simulink model "WormAndGearConstraint"  (R2024a)
settings: Solver=ode45  StartTime=0.0  StopTime=120  MaxStep=0.01  RelTol=1e-3
PreLoadFcn:
  | addpath(fullfile('WormAndGearConstraintSupport','Data'));
  | addpath(fullfile('WormAndGearConstraintSupport','Scripts'));
model workspace: external: MATLAB File WormAndGearConstraintParameters.m (data not in the file)
undefined symbols (not defined in the file or in its folder): slewdrive, X, Y, Z
libraries: sm_lib x75, neural x40, nesl_utility x38, fl_lib x32, WormAndGearConstraintLibrary x24, ee_lib x6, slpidlib x6, spsSeriesRLCBranchLib x2, fl_ps_legacy_lib x1, spsPWMGeneratorDCDCLib x1, spsMosfetLib x1, spsPVArrayLib x1
(part 1 of 6)
CloseFcn:
  | rmpath(fullfile('WormAndGearConstraintSupport','Data'));
  | rmpath(fullfile('WormAndGearConstraintSupport','Scripts'));
Description:
  | Using the Worm and Gear Constraint Block - Solar Tracker
settings Model: SimulationMode=accelerator  Creator=The MathWorks, Inc.  LastModifiedBy=Kshitij Shetty
settings SolverCC: AlgebraicLoopSolver=TrustRegion
settings DataIOCC: ReturnWorkspaceOutputs=off
settings OptimizationCC: ReuseModelBlockBuffer=off
settings DebuggingCC: UnconnectedInputMsg=warning  UnconnectedOutputMsg=warning  UnconnectedLineMsg=warning  SubsystemReferenceDiagnosticForUnitTest=warning  ArithmeticOperatorsInVariantConditions=warning
settings ModelReferenceCC: EnableRefExpFcnMdlSchedulingChecks=on
settings SFSimCC: SimUseLocalCustomCode=off  CustomCodeUndefinedFunction=UseInterfaceOnly
settings RTWCC: RTWUseLocalCustomCode=off  GPUComputeCapability=3.5
settings CodeAppCC: StateflowObjectComments=on
settings ConfigComp: CovMetricSettings=dswe
settings SimscapeCC: SimscapeNormalizeSystem=off  SimscapeNominalValues="[{\"value\":\"10\",\"unit\":\"V\"},{\"value\":\"1\",\"unit\":\"A\"},{\"value\":\"10\",\"unit\":\"N*m\"},{\"value\":\"10\",\"unit\":\"bar\"},{\"value\":\"100\",\"unit\":\"kJ/kg\"},{\"value\":\"1\",\"unit\":\"kW\"},{\"value\":\"300\",\"unit\":\"K\"},{\"value\":\"100\",\"unit\":\"cm^3/s\"},{\"value\":\"1\",\"unit\":\"kN\"},{\"value\":\"1\",\"unit\":\"g/cm^3\"},{\"value\":\"1\",\"unit\":\"l\"},{\"value\":\"1\",\"unit\":\"cm^2\"},{\"value\":\"60\",\"unit\":\"Hz\"}]"  SimscapeLogType=all  SimscapeLogSimulationStatistics=on  SimscapeLogName=simlogWormAndGearConstraint
settings DiagnosticsConfigSet: SimMechanicsUnconnectedFramePorts=none
settings ExplorerConfigSet: InternalSimMechanicsExplorerSettings="<ExplorerConfiguration><canonicalview>default</canonicalview><AnimationSetting><BasePlaybackSpeed>1.0</BasePlaybackSpeed><PlaybackSpeedFactor>2.0</PlaybackSpeedFactor></AnimationSetting><TilePanel><TileInfo><Tiles Columns=\"1\" Count=\"2\" Rows=\"2\"><Column Weight=\"1\"/><Row Weight=\"0.499\"/><Row Weight=\"0.501\"/><Tile Height=\"1\" Width=\"1\" X=\"0\" Y=\"0\"/><Tile Height=\"1\" Width=\"1\" X=\"0\" Y=\"1\"/></Tiles></TileInfo><SceneInfo><SceneViewer><BGColor><R>0.60000002384185791</R><G>0.60000002384185791</G><B>0.60000002384185791</B></BGColor><Camera><DoPerspective>off</DoPerspective><Position><X>1.57222703754827808</X><Y>0.0360261259505583187</Y><Z>2.51324508298032256</Z></Position><Center><X>0.0305976255689774934</X><Y>1.57765553792985891</Y><Z>0.971615671001021308</Z></Center><Up><X>-0.408248290463863073</X><Y>0.408248290463863073</Y><Z>0.816496580927726145</Z></Up><ViewLimDist>1</ViewLimDist><YLim>1.55175099611282352</YLim><XLim>5.69835401422903765</XLim></Camera></SceneViewer><SceneViewer><BGColor><R>0.60000002384185791</R><G>0.60000002384185791</G><B>0.60000002384185791</B></BGColor><Camera><DoPerspective>on</DoPerspective><Position><X>0.0528984487695908223</X><Y>3.2815089600888423</Y><Z>1.01068686751161962</Z></Position><Center><X>-0.0110921743538067302</X><Y>3.04874647132397136</Y><Z>0.949794701859282609</Z></Center><Up><X>-0.0543238299990527959</X><Y>-0.238711140095184626</Y><Z>0.969569962967444243</Z></Up><ViewLimDist>1</ViewLimDist><YLim>0.466307658154998583</YLim><XLim>1.70832142063418924</XLim></Camera></SceneViewer></SceneInfo></TilePanel><MechEditorPanel><Cameras><Camera><Id>Camera1</Id><Value><Name>Slew Drive View</Name><NativeCamera><PositionKeyframeSet><Keyframe><Time>0</Time><Value><X>0.052898448769590822</X><Y>3.2815089600888423</Y><Z>1.0106868675116196</Z></Value></Keyframe></PositionKeyframeSet><CenterKeyframeSet><Keyframe><Time>0</Time><Value><X>-0.01109217435380673</X><Y>3.0487464713239714</Y><Z>0.94979470185928261</Z></Value></Keyframe></CenterKeyframeSet><UpVectorKeyframeSet><Keyframe><Time>0</Time><Value><X>-0.054323829999052796</X><Y>-0.23871114009518463</Y><Z>0.96956996296744424</Z></Value></Keyframe></UpVectorKeyframeSet></NativeCamera></Value></Camera></Cameras><GfxPanelCameraMap><MapElement CameraMLId=\"Camera1\" GfxPanelIndex=\"1\"/></GfxPanelCameraMap><VideoCreator><PlaybackSpeedRatio>2.0</PlaybackSpeedRatio><FrameRate>30</FrameRate><VideoFormat>Motion JPEG AVI</VideoFormat><FrameSize>auto</FrameSize></VideoCreator></MechEditorPanel></ExplorerConfiguration>"

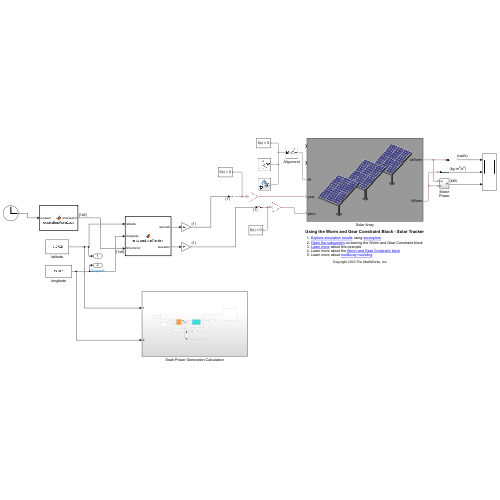
[thumbnail: Simulink's stored preview of the top-level diagram]
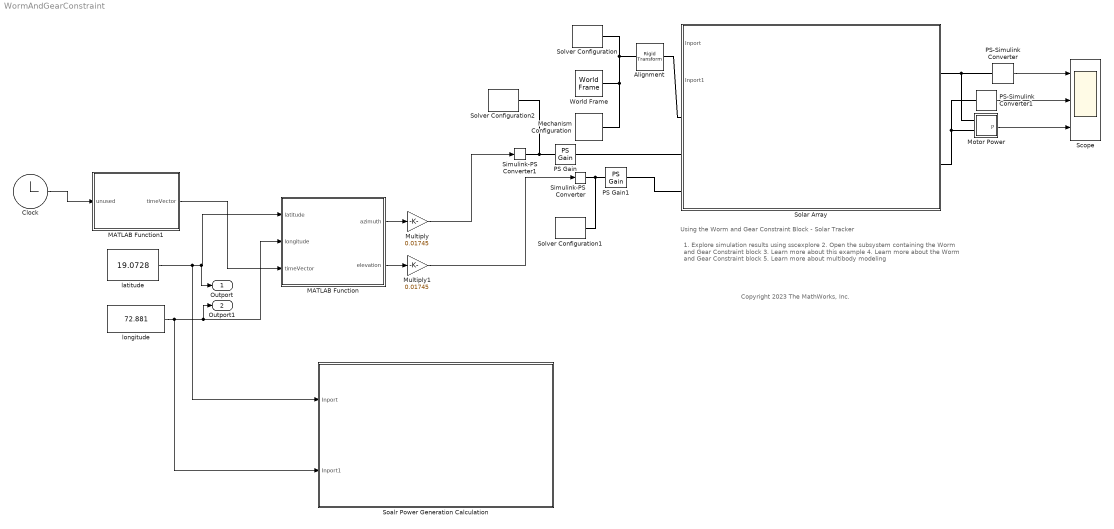
== system WormAndGearConstraint ==
  note: Copyright 2023 The MathWorks, Inc.
  note: Using the Worm and Gear Constraint Block - Solar Tracker
  note: 1. Explore simulation results using sscexplore
      | 2. Open the subsystem containing the Worm and Gear Constraint block
      | 3. Learn more about this example
      | 4. Learn more about the Worm and Gear Constraint block
      | 5. Learn more about multibody modeling
  Alignment : sm_lib/Frames and Transforms/Rigid Transform  RotationMethod=AlignedAxes  FollAlignAxisA=+Z  BaseAlignAxisA=+Z  FollAlignAxisB=+Y  BaseAlignAxisB=-X  RotationStandardAxis=+Z  RotationAngle=0.0  RotationAngleUnits=deg  RotationArbitraryAxis=[0 0 1]  RotationSequenceAxes=FollowerAxes  RotationSequence=XYX  RotationSequenceAngles=[0 0 0]  RotationSequenceAnglesUnits=deg  RotationMatrix=[1 0 0; 0 1 0; 0 0 1]  Quaternion=[1 0 0 0]  TranslationMethod=None  TranslationCartesianOffset=[0 0 0]  TranslationCartesianOffsetUnits=m  TranslationStandardAxis=+Z  TranslationStandardOffset=0  TranslationStandardOffsetUnits=m  TranslationROffset=0  TranslationROffsetUnits=m  TranslationThetaOffset=0  TranslationThetaOffsetUnits=deg  TranslationZOffset=0  TranslationZOffsetUnits=m
  Clock : Clock
  MATLAB Function : MATLAB Function  TreatAsAtomicUnit=on
  MATLAB Function1 : MATLAB Function  TreatAsAtomicUnit=on
  Mechanism Configuration : sm_lib/Utilities/Mechanism Configuration  UniformGravity=Constant  GravityVector=[0 0 -9.80665]  GravityVectorUnits=m/s^2  LinearizationDelta=0.001  JointModeTransitionNonlinearIterations=2
  Motor Power : Subsystem
  Multiply : Gain  Gain=0.01745
  Multiply1 : Gain  Gain=0.01745
  PS Gain : fl_lib/Physical Signals/Functions/PS Gain  gain=1
  PS Gain1 : fl_lib/Physical Signals/Functions/PS Gain  gain=1
  PS-Simulink Converter : nesl_utility/PS-Simulink Converter  PhysicalDomain=network_engine_domain  SubClassName=ps_output  LeftPortType=input  RightPortType=output  PseudoPeriodic=off  Frequencies=[]  VectorFormat=inherit  Unit=inherit  AffineConversion=off
  PS-Simulink Converter1 : nesl_utility/PS-Simulink Converter  PhysicalDomain=network_engine_domain  SubClassName=ps_output  LeftPortType=input  RightPortType=output  PseudoPeriodic=off  Frequencies=[]  VectorFormat=inherit  Unit=inherit  AffineConversion=off
  Scope : Scope  NumInputPorts=3
  Simulink-PS Converter : nesl_utility/Simulink-PS Converter  PhysicalDomain=network_engine_domain  SubClassName=ps_input  LeftPortType=input  RightPortType=output  PseudoPeriodic=off  Frequencies=[]  NoiseDistribution=none  NoiseParameters=[]  Unit=1  AffineConversion=off  FilteringAndDerivatives=provide  SimscapeFilterOrder=1  InputFilterTimeConstant=0.001  UdotUserProvided=0
  Simulink-PS Converter1 : nesl_utility/Simulink-PS Converter  PhysicalDomain=network_engine_domain  SubClassName=ps_input  LeftPortType=input  RightPortType=output  PseudoPeriodic=off  Frequencies=[]  NoiseDistribution=none  NoiseParameters=[]  Unit=1  AffineConversion=off  FilteringAndDerivatives=provide  SimscapeFilterOrder=1  InputFilterTimeConstant=0.001  UdotUserProvided=0
  Soalr Power Generation Calculation : Subsystem
  Solar Array : Subsystem
      mask Display:
      | image(fullfile('WormAndGearConstraintSupport','Images','SolarArray.png'));
      | port_label('lconn',1,'W');
      | port_label('lconn',2,'yaw');
      | port_label('lconn',3,'pitch');
      | port_label('rconn',1,'wWorm');
      | port_label('rconn',2,'tWorm');
  Solver Configuration : nesl_utility/Solver Configuration  PhysicalDomain=network_engine_domain  SubClassName=solver  LeftPortType=input  RightPortType=generic  Tones=[]  Harmonics=[]  SimulateNoise=off  Profile=off  UseLocalSampling=off  EnableSwitchedLinearOptims=on  FrequencyDomain=off  UseCCode=off  RelTol=0.001  AbsTol=1e-06  MinStep=1e-09  ToWorkspace=off  RevertToSquareIcSolve=off  NumHomotopyIterations=100  PhasorMode=off  PhasorModeNumHarmonics=1  ConsistencySolver=NEWTON_FTOL  IndexReductionMethod=DerivativeReplacement  DoDC=off  ResidualTolerance=1e-09  ConsistencyTolSource=GLOBAL  ConsistencyAbsTol=0.001  ConsistencyRelTol=0.001  ConsistencyTolFactor=0.001  UseLocalSolver=off  LocalSolverChoice=NE_BACKWARD_EULER_ADVANCER  ResolveIndetEquations=on  FunctionEvalNumThread=1  LocalSolverSampleTime=0.001  DoFixedCost=off  MaxNonlinIter=3  MaxModeIter=2  ComputeImpulses=off  ImpulseIterations=2  LinearAlgebra=Sparse  LinearAlgebraNumThread=0  EquationFormulation=NE_TIME_EF  DelaysMemoryBudget=1024  AutomaticFiltering=on  FilteringTimeConstant=0.001  PartitionStorageMethod=AS_NEEDED  PartitionMemoryBudget=1024  PartitionMethod=FAST  MultibodyUseLocalSolver=off  MultibodyLocalSolverChoice=ODE1  MultibodyLocalSolverSampleTime=0.001
  Solver Configuration1 : nesl_utility/Solver Configuration  PhysicalDomain=network_engine_domain  SubClassName=solver  LeftPortType=input  RightPortType=generic  Tones=[]  Harmonics=[]  SimulateNoise=off  Profile=off  UseLocalSampling=off  EnableSwitchedLinearOptims=on  FrequencyDomain=off  UseCCode=off  RelTol=0.001  AbsTol=1e-06  MinStep=1e-09  ToWorkspace=off  RevertToSquareIcSolve=off  NumHomotopyIterations=100  PhasorMode=off  PhasorModeNumHarmonics=1  ConsistencySolver=NEWTON_FTOL  IndexReductionMethod=DerivativeReplacement  DoDC=off  ResidualTolerance=1e-09  ConsistencyTolSource=GLOBAL  ConsistencyAbsTol=0.001  ConsistencyRelTol=0.001  ConsistencyTolFactor=0.001  UseLocalSolver=off  LocalSolverChoice=NE_BACKWARD_EULER_ADVANCER  ResolveIndetEquations=on  FunctionEvalNumThread=1  LocalSolverSampleTime=0.001  DoFixedCost=off  MaxNonlinIter=3  MaxModeIter=2  ComputeImpulses=off  ImpulseIterations=2  LinearAlgebra=Sparse  LinearAlgebraNumThread=0  EquationFormulation=NE_TIME_EF  DelaysMemoryBudget=1024  AutomaticFiltering=on  FilteringTimeConstant=0.001  PartitionStorageMethod=AS_NEEDED  PartitionMemoryBudget=1024  PartitionMethod=FAST  MultibodyUseLocalSolver=off  MultibodyLocalSolverChoice=ODE1  MultibodyLocalSolverSampleTime=0.001
  Solver Configuration2 : nesl_utility/Solver Configuration  PhysicalDomain=network_engine_domain  SubClassName=solver  LeftPortType=input  RightPortType=generic  Tones=[]  Harmonics=[]  SimulateNoise=off  Profile=off  UseLocalSampling=off  EnableSwitchedLinearOptims=on  FrequencyDomain=off  UseCCode=off  RelTol=0.001  AbsTol=1e-06  MinStep=1e-09  ToWorkspace=off  RevertToSquareIcSolve=off  NumHomotopyIterations=100  PhasorMode=off  PhasorModeNumHarmonics=1  ConsistencySolver=NEWTON_FTOL  IndexReductionMethod=DerivativeReplacement  DoDC=off  ResidualTolerance=1e-09  ConsistencyTolSource=GLOBAL  ConsistencyAbsTol=0.001  ConsistencyRelTol=0.001  ConsistencyTolFactor=0.001  UseLocalSolver=off  LocalSolverChoice=NE_BACKWARD_EULER_ADVANCER  ResolveIndetEquations=on  FunctionEvalNumThread=1  LocalSolverSampleTime=0.001  DoFixedCost=off  MaxNonlinIter=3  MaxModeIter=2  ComputeImpulses=off  ImpulseIterations=2  LinearAlgebra=Sparse  LinearAlgebraNumThread=0  EquationFormulation=NE_TIME_EF  DelaysMemoryBudget=1024  AutomaticFiltering=on  FilteringTimeConstant=0.001  PartitionStorageMethod=AS_NEEDED  PartitionMemoryBudget=1024  PartitionMethod=FAST  MultibodyUseLocalSolver=off  MultibodyLocalSolverChoice=ODE1  MultibodyLocalSolverSampleTime=0.001
  World Frame : sm_lib/Frames and Transforms/World Frame
  latitude : Constant  Value=19.0728
  longitude : Constant  Value=72.881
  Outport : Outport
  Outport1 : Outport  Port=2
  wires:
  PS-Simulink Converter1/1 -> Scope/2
  PS-Simulink Converter/1 -> Scope/1
  Motor Power/1(P) -> Scope/3
  latitude/1 -> Soalr Power Generation Calculation/1(Inport), Outport/1, MATLAB Function/1(latitude)
  MATLAB Function1/1(timeVector) -> MATLAB Function/3(timeVector)
  Clock/1 -> MATLAB Function1/1(unused)
  longitude/1 -> Soalr Power Generation Calculation/2(Inport1), Outport1/1, MATLAB Function/2(longitude)
  MATLAB Function/1(azimuth) -> Multiply/1
  Multiply/1 -> Simulink-PS Converter1/1
  MATLAB Function/2(elevation) -> Multiply1/1
  Multiply1/1 -> Simulink-PS Converter/1
  connections:
  World Frame/RConn1 -- Solver Configuration/RConn1 -- Alignment/LConn1 -- Mechanism Configuration/RConn1
  Alignment/RConn1 -- Solar Array/LConn1
  PS-Simulink Converter/LConn1 -- Motor Power/LConn1 -- Solar Array/RConn1
  PS-Simulink Converter1/LConn1 -- Motor Power/LConn2 -- Solar Array/RConn2
  Simulink-PS Converter/RConn1 -- Solver Configuration1/RConn1 -- PS Gain1/LConn1
  PS Gain1/RConn1 -- Solar Array/LConn3
  PS Gain/LConn1 -- Solver Configuration2/RConn1 -- Simulink-PS Converter1/RConn1
  PS Gain/RConn1 -- Solar Array/LConn2

== system WormAndGearConstraint/Motor Power ==
  Motor Power : fl_ps_legacy_lib/Legacy Physical Signals/Functions/PS Product
  PS-Simulink Converter2 : nesl_utility/PS-Simulink Converter  PhysicalDomain=network_engine_domain  SubClassName=ps_output  LeftPortType=input  RightPortType=output  PseudoPeriodic=off  Frequencies=[]  VectorFormat=1-D array  Unit=kW  AffineConversion=off
  w : PMIOPort  Side=Left
  t : PMIOPort  Port=2  Side=Left
  P : Outport
  wires:
  PS-Simulink Converter2/1 -> P/1
  connections:
  PS-Simulink Converter2/LConn1 -- Motor Power/RConn1
  Motor Power/LConn2 -- t/RConn1
  Motor Power/LConn1 -- w/RConn1

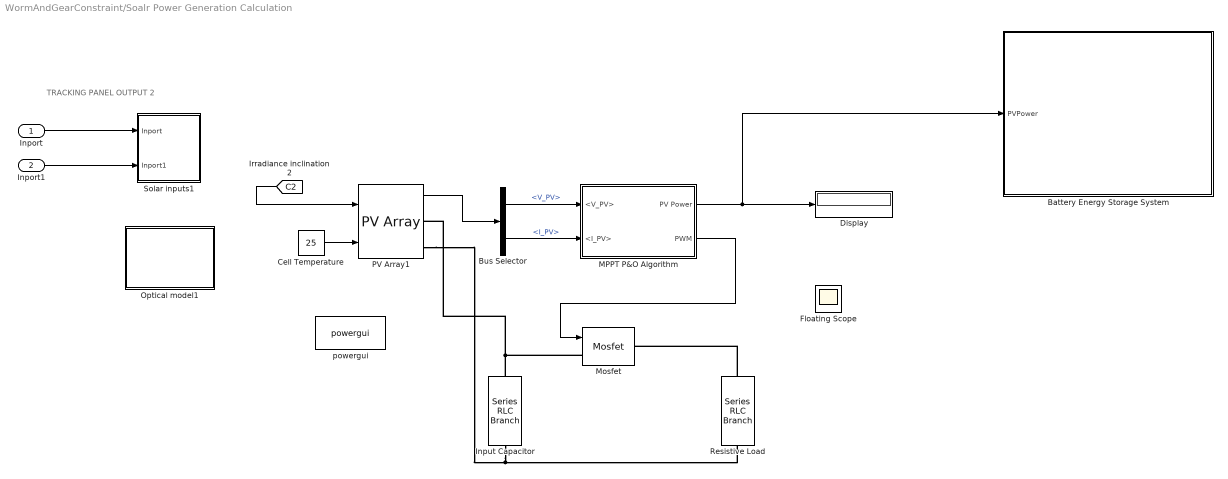
== system WormAndGearConstraint/Soalr Power Generation Calculation ==
  note: TRACKING PANEL OUTPUT 2
  Inport : Inport
  Inport1 : Inport  Port=2
  Battery Energy Storage System : Subsystem
  Bus Selector : BusSelector  OutputSignals=V_PV,I_PV
  Cell Temperature : Constant  Value=25
  Display : Display
  Floating Scope : Scope
      settings: Floating=on
  Input Capacitor : spsSeriesRLCBranchLib/Series RLC Branch  LConnTagsString=__new0  RConnTagsString=__new0  BranchType=C  Resistance=10  Inductance=1e-3  SetiL0=off  InitialCurrent=0  Capacitance=1000e-6  Setx0=off  InitialVoltage=0  Measurements=None
  MPPT P&O Algorithm : Subsystem  mask(MPPT Perturb and Observe Algorithm Block){Fsw=1000, StepSize=1e-6}
      mask prompts: Fsw "PWM Switching frequency (Hz):"; StepSize "PWM Duty Cycle (delta) Step Size"
      mask help:
      | MPPT Perturb & Observe Algorithm Block
      | Developed by Rodney Tan (PhD)
      | Version 1.00 Sep 2019
      |
      | This block perform photovoltaic panel Maximum Power Point Tracking based on Perturb & Observe algorithm.
      | This MPPT P&O method is implemented using basic Simulink block only.
      | This MPPT block take in Voltage and Current from photovoltaic panel and output PWM switching signal to drive the DC converter
      mask Help:
      | <b><u>Block Setting</u></b>
      | <b>PWM Switching Frequency (Hz)</b>
      | Specify the PWM switching frequency in Hz.
      | 
      | <b>PWM Duty Cycle Step Size</b>
      | Specify the PWM duty cycle (delta) step size. Default value is 1e-6.
      mask TypeOptions Fsw:
      | PWM Generator
      | (DC-DC)/Fsw
  Mosfet : spsMosfetLib/Mosfet  Ron=0.1  Lon=0  Rd=0.01  Vfd=0  IC=0  Rs=1e5  Cs=inf  Measurements=off
  Optical model1 : Subsystem
  PV Array1 : spsPVArrayLib/PV Array  Npar=1  Nser=3  PlotType=array @ 1000 W/m2 & specified temperatures  S_vec="[ 1000  500  100 ]"  Temp_C_vec="[ 45 25  ]"  ModuleName=A10Green Technology A10J-M60-240  PlotWhenSelected=off  Pm=240.5376  Ncell=60  Voc=36.84  Isc=8.32  Vm=30.72  Im=7.83  beta_Voc_pc=-0.359  alpha_Isc_pc=0.096995  beta_Voc=-0.13226  alpha_Isc=0.00807  IL=8.3299  I0=2.8736e-10  nI=0.99259  Rsh=330.6558  Rs=0.19366  RobustModel=off  RobustCellTemperature=25  BAL=on  Tc=1e-6  Tfilter=5e-5
  Resistive Load : spsSeriesRLCBranchLib/Series RLC Branch  LConnTagsString=__new0  RConnTagsString=__new0  BranchType=R  Resistance=5  Inductance=1e-3  SetiL0=off  InitialCurrent=0  Capacitance=1e-6  Setx0=off  InitialVoltage=0  Measurements=None
  Solar inputs1 : Subsystem
  powergui : sps_lib/powergui  Priority=1  SimulationMode=Discrete  SampleTime=1e-5  frequency=60  Iterations=50  frequencyindice=0  Pbase=100e6  ErrMax=1e-4  UnitsV=kV  UnitsW=MW  buscounter=0  FunctionMessages=off  echomessages=off  EnableUseOfTLC=off  CurrentSourceSwitches=off  DisableSnubberDevices=off  DisableRonSwitches=off  DisableVfSwitches=off  DisplayEquations=off  AutomaticDiscreteSolvers=off  SolverType=Tustin/Backward Euler (TBE)  Interpol=off  ExternalGateDelay=off  methode=off  Ts=100  x0status=blocks  SPID=off  SwTol=0  HookPort=off  NonlinearTolerance=1e-4  nMaxIteration=100  ContinueOnMaxIteration=off  RestoreLinks=warning  ResistiveCurrentMeasurement=off  Frange=[0:2:500]  Ylog=off  Xlog=on  ShowGrid=off  save=off  variable=ZData  structure=0  ZoomFFT=off  StartTime=0.0  cycles=1  DisplayStyle=1  fundamental=60  FreqAxis=off  MaxFrequency=1000  frequencyindicesteady=1  RmsSteady=1  display=off
  wires:
  Bus Selector/1 -> MPPT P&O Algorithm/1(<V_PV>)  "<V_PV>"
  PV Array1/1 -> Bus Selector/1
  Cell Temperature/1 -> PV Array1/2
  Bus Selector/2 -> MPPT P&O Algorithm/2(<I_PV>)  "<I_PV>"
  MPPT P&O Algorithm/2(PWM) -> Mosfet/1
  MPPT P&O Algorithm/1(PV Power) -> Battery Energy Storage System/1(PVPower), Display/1
  [C2] -> PV Array1/1
  Inport/1 -> Solar inputs1/1(Inport)
  Inport1/1 -> Solar inputs1/2(Inport1)
  connections:
  PV Array1/RConn1 -- Mosfet/LConn1 -- Input Capacitor/LConn1
  Resistive Load/LConn1 -- Mosfet/RConn1
  PV Array1/RConn2 -- Resistive Load/RConn1 -- Input Capacitor/RConn1

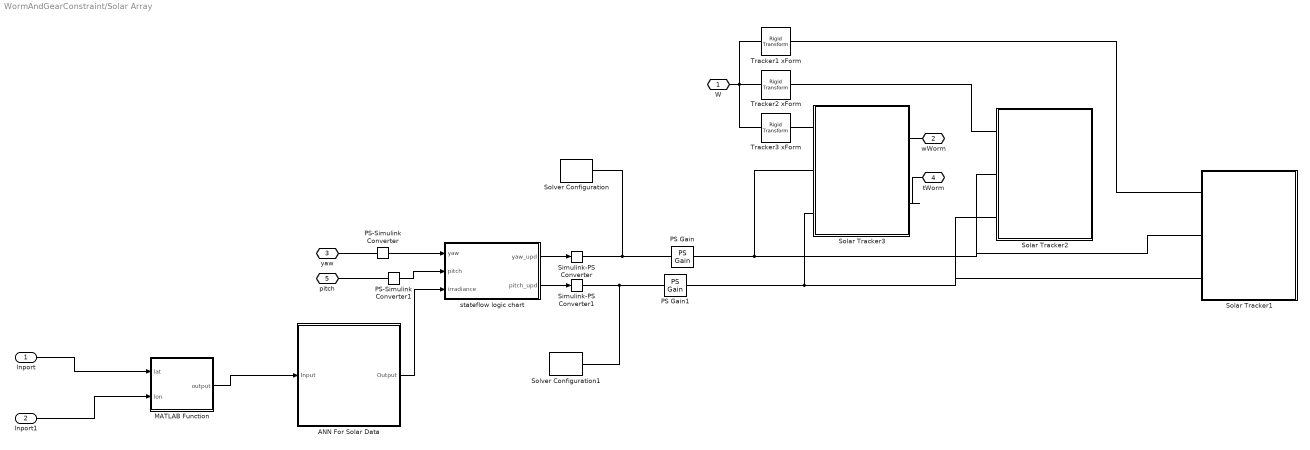
== system WormAndGearConstraint/Solar Array ==
  Inport : Inport
  Inport1 : Inport  Port=2
  ANN For Solar Data : Subsystem
      mask help: Function Fitting Neural Network
      mask Display: e = 0.06;c1 = [120 150 230]/255;c2 = ([120 150 230]+0)/383;c3 = ([120 150 230]+128)/383;patch([0 1 1 0],[0 0 1 1],c1);patch([0 1 1 1-e 1-e 0+e],[0 0 1 1-e 0+e 0+e],c2);patch([0 0 1 1-e 0+e 0+e],[0 1 1 1-e 1-e 0+e],c3);plot([0 1 1 0 0],[0 0 1 1 0]);fprintf('NNET');port_label('input',1,' Input');port_label('output',1,'Output ');
  MATLAB Function : MATLAB Function  TreatAsAtomicUnit=on
  PS Gain : fl_lib/Physical Signals/Functions/PS Gain  gain=1
  PS Gain1 : fl_lib/Physical Signals/Functions/PS Gain  gain=1
  PS-Simulink Converter : nesl_utility/PS-Simulink Converter  PhysicalDomain=network_engine_domain  SubClassName=ps_output  LeftPortType=input  RightPortType=output  PseudoPeriodic=off  Frequencies=[]  VectorFormat=inherit  Unit=inherit  AffineConversion=off
  PS-Simulink Converter1 : nesl_utility/PS-Simulink Converter  PhysicalDomain=network_engine_domain  SubClassName=ps_output  LeftPortType=input  RightPortType=output  PseudoPeriodic=off  Frequencies=[]  VectorFormat=inherit  Unit=inherit  AffineConversion=off
  Simulink-PS Converter : nesl_utility/Simulink-PS Converter  PhysicalDomain=network_engine_domain  SubClassName=ps_input  LeftPortType=input  RightPortType=output  PseudoPeriodic=off  Frequencies=[]  NoiseDistribution=none  NoiseParameters=[]  Unit=1  AffineConversion=off  FilteringAndDerivatives=provide  SimscapeFilterOrder=1  InputFilterTimeConstant=0.001  UdotUserProvided=0
  Simulink-PS Converter1 : nesl_utility/Simulink-PS Converter  PhysicalDomain=network_engine_domain  SubClassName=ps_input  LeftPortType=input  RightPortType=output  PseudoPeriodic=off  Frequencies=[]  NoiseDistribution=none  NoiseParameters=[]  Unit=1  AffineConversion=off  FilteringAndDerivatives=provide  SimscapeFilterOrder=1  InputFilterTimeConstant=0.001  UdotUserProvided=0
  Solar Tracker1 : Subsystem
      mask Display:
      | image(fullfile('WormAndGearConstraintSupport','Images','SolarTracker.png'));
      | port_label('lconn',1,'B');
      | port_label('lconn',2,'y');
      | port_label('lconn',3,'p');
  Solar Tracker2 : Subsystem
      mask Display:
      | image(fullfile('WormAndGearConstraintSupport','Images','SolarTracker.png'));
      | port_label('lconn',1,'B');
      | port_label('lconn',2,'y');
      | port_label('lconn',3,'p');
  Solar Tracker3 : Subsystem
      mask Display:
      | image(fullfile('WormAndGearConstraintSupport','Images','SolarTracker.png'));
      | port_label('lconn',1,'B');
      | port_label('lconn',2,'y');
      | port_label('lconn',3,'p');
      | port_label('rconn',1,'w');
      | port_label('rconn',2,'t');
  Solver Configuration : nesl_utility/Solver Configuration  PhysicalDomain=network_engine_domain  SubClassName=solver  LeftPortType=input  RightPortType=generic  Tones=[]  Harmonics=[]  SimulateNoise=off  Profile=off  UseLocalSampling=off  EnableSwitchedLinearOptims=on  FrequencyDomain=off  UseCCode=off  RelTol=0.001  AbsTol=0.001  MinStep=1e-09  ToWorkspace=off  RevertToSquareIcSolve=off  NumHomotopyIterations=100  PhasorMode=off  PhasorModeNumHarmonics=1  ConsistencySolver=NEWTON_XTOL_AFTER_FTOL  IndexReductionMethod=DerivativeReplacement  DoDC=off  ResidualTolerance=1e-09  ConsistencyTolSource=GLOBAL  ConsistencyAbsTol=0.001  ConsistencyRelTol=0.001  ConsistencyTolFactor=0.001  UseLocalSolver=off  LocalSolverChoice=NE_BACKWARD_EULER_ADVANCER  ResolveIndetEquations=on  FunctionEvalNumThread=1  LocalSolverSampleTime=0.001  DoFixedCost=off  MaxNonlinIter=3  MaxModeIter=2  ComputeImpulses=off  ImpulseIterations=2  LinearAlgebra=auto  LinearAlgebraNumThread=0  EquationFormulation=NE_TIME_EF  DelaysMemoryBudget=1024  AutomaticFiltering=on  FilteringTimeConstant=0.001  PartitionStorageMethod=AS_NEEDED  PartitionMemoryBudget=1024  PartitionMethod=ROBUST  MultibodyUseLocalSolver=off  MultibodyLocalSolverChoice=ODE1  MultibodyLocalSolverSampleTime=0.001
  Solver Configuration1 : nesl_utility/Solver Configuration  PhysicalDomain=network_engine_domain  SubClassName=solver  LeftPortType=input  RightPortType=generic  Tones=[]  Harmonics=[]  SimulateNoise=off  Profile=off  UseLocalSampling=off  EnableSwitchedLinearOptims=on  FrequencyDomain=off  UseCCode=off  RelTol=0.001  AbsTol=0.001  MinStep=1e-09  ToWorkspace=off  RevertToSquareIcSolve=off  NumHomotopyIterations=100  PhasorMode=off  PhasorModeNumHarmonics=1  ConsistencySolver=NEWTON_XTOL_AFTER_FTOL  IndexReductionMethod=DerivativeReplacement  DoDC=off  ResidualTolerance=1e-09  ConsistencyTolSource=GLOBAL  ConsistencyAbsTol=0.001  ConsistencyRelTol=0.001  ConsistencyTolFactor=0.001  UseLocalSolver=off  LocalSolverChoice=NE_BACKWARD_EULER_ADVANCER  ResolveIndetEquations=on  FunctionEvalNumThread=1  LocalSolverSampleTime=0.001  DoFixedCost=off  MaxNonlinIter=3  MaxModeIter=2  ComputeImpulses=off  ImpulseIterations=2  LinearAlgebra=auto  LinearAlgebraNumThread=0  EquationFormulation=NE_TIME_EF  DelaysMemoryBudget=1024  AutomaticFiltering=on  FilteringTimeConstant=0.001  PartitionStorageMethod=AS_NEEDED  PartitionMemoryBudget=1024  PartitionMethod=ROBUST  MultibodyUseLocalSolver=off  MultibodyLocalSolverChoice=ODE1  MultibodyLocalSolverSampleTime=0.001
  Tracker1 xForm : sm_lib/Frames and Transforms/Rigid Transform  RotationMethod=None  FollAlignAxisA=+X  BaseAlignAxisA=+Y  FollAlignAxisB=+Y  BaseAlignAxisB=+Z  RotationStandardAxis=+Z  RotationAngle=0.0  RotationAngleUnits=deg  RotationArbitraryAxis=[0 0 1]  RotationSequenceAxes=FollowerAxes  RotationSequence=XYX  RotationSequenceAngles=[0 0 0]  RotationSequenceAnglesUnits=deg  RotationMatrix=[1 0 0; 0 1 0; 0 0 1]  Quaternion=[1 0 0 0]  TranslationMethod=Cartesian  TranslationCartesianOffset=tracker1_offset  TranslationCartesianOffsetUnits=m  TranslationStandardAxis=+Z  TranslationStandardOffset=0  TranslationStandardOffsetUnits=m  TranslationROffset=0  TranslationROffsetUnits=m  TranslationThetaOffset=0  TranslationThetaOffsetUnits=deg  TranslationZOffset=0  TranslationZOffsetUnits=m
  Tracker2 xForm : sm_lib/Frames and Transforms/Rigid Transform  RotationMethod=None  FollAlignAxisA=+Z  BaseAlignAxisA=+Z  FollAlignAxisB=+Y  BaseAlignAxisB=-X  RotationStandardAxis=+Z  RotationAngle=0.0  RotationAngleUnits=deg  RotationArbitraryAxis=[0 0 1]  RotationSequenceAxes=FollowerAxes  RotationSequence=XYX  RotationSequenceAngles=[0 0 0]  RotationSequenceAnglesUnits=deg  RotationMatrix=[1 0 0; 0 1 0; 0 0 1]  Quaternion=[1 0 0 0]  TranslationMethod=Cartesian  TranslationCartesianOffset=tracker2_offset  TranslationCartesianOffsetUnits=m  TranslationStandardAxis=+Z  TranslationStandardOffset=0  TranslationStandardOffsetUnits=m  TranslationROffset=0  TranslationROffsetUnits=m  TranslationThetaOffset=0  TranslationThetaOffsetUnits=deg  TranslationZOffset=0  TranslationZOffsetUnits=m
  Tracker3 xForm : sm_lib/Frames and Transforms/Rigid Transform  RotationMethod=None  FollAlignAxisA=+X  BaseAlignAxisA=+Y  FollAlignAxisB=+Y  BaseAlignAxisB=+Z  RotationStandardAxis=+Z  RotationAngle=0.0  RotationAngleUnits=deg  RotationArbitraryAxis=[0 0 1]  RotationSequenceAxes=FollowerAxes  RotationSequence=XYX  RotationSequenceAngles=[0 0 0]  RotationSequenceAnglesUnits=deg  RotationMatrix=[1 0 0; 0 1 0; 0 0 1]  Quaternion=[1 0 0 0]  TranslationMethod=Cartesian  TranslationCartesianOffset=tracker3_offset  TranslationCartesianOffsetUnits=m  TranslationStandardAxis=+Z  TranslationStandardOffset=0  TranslationStandardOffsetUnits=m  TranslationROffset=0  TranslationROffsetUnits=m  TranslationThetaOffset=0  TranslationThetaOffsetUnits=deg  TranslationZOffset=0  TranslationZOffsetUnits=m
  stateflow logic chart : Stateflow chart  TreatAsAtomicUnit=on
  W : PMIOPort  Side=Left
  wWorm : PMIOPort  Port=2  Side=Right
  yaw : PMIOPort  Port=3  Side=Left
  tWorm : PMIOPort  Port=4  Side=Right
  pitch : PMIOPort  Port=5  Side=Left
  wires:
  stateflow logic chart/1(yaw_upd) -> Simulink-PS Converter/1
  stateflow logic chart/2(pitch_upd) -> Simulink-PS Converter1/1
  PS-Simulink Converter1/1 -> stateflow logic chart/2(pitch)
  PS-Simulink Converter/1 -> stateflow logic chart/1(yaw)
  MATLAB Function/1(output) -> ANN For Solar Data/1(Input)
  ANN For Solar Data/1(Output) -> stateflow logic chart/3(irradiance)
  Inport/1 -> MATLAB Function/1(lat)
  Inport1/1 -> MATLAB Function/2(lon)
  connections:
  Tracker3 xForm/LConn1 -- Tracker1 xForm/LConn1 -- W/RConn1 -- Tracker2 xForm/LConn1
  Tracker3 xForm/RConn1 -- Solar Tracker3/LConn1
  Solar Tracker3/RConn2 -- tWorm/RConn1
  Solar Tracker3/RConn1 -- wWorm/RConn1
  Tracker2 xForm/RConn1 -- Solar Tracker2/LConn1
  Tracker1 xForm/RConn1 -- Solar Tracker1/LConn1
  yaw/RConn1 -- PS-Simulink Converter/LConn1
  pitch/RConn1 -- PS-Simulink Converter1/LConn1
  Simulink-PS Converter/RConn1 -- Solver Configuration/RConn1 -- PS Gain/LConn1
  PS Gain/RConn1 -- Solar Tracker1/LConn2 -- Solar Tracker2/LConn2 -- Solar Tracker3/LConn2
  PS Gain1/RConn1 -- Solar Tracker1/LConn3 -- Solar Tracker2/LConn3 -- Solar Tracker3/LConn3
  Simulink-PS Converter1/RConn1 -- Solver Configuration1/RConn1 -- PS Gain1/LConn1

== system WormAndGearConstraint/Soalr Power Generation Calculation/Battery Energy Storage System ==
  PVPower : Inport
  Constant : Constant  Value=100
  Constant1 : Constant
  Constant2 : Constant  Value=400
  Constant3 : Constant  Value=400
  Integrator : Integrator  InitialCondition=0.5
  MATLAB Function : MATLAB Function  TreatAsAtomicUnit=on
  MATLAB Function1 : MATLAB Function  TreatAsAtomicUnit=on
  MATLAB Function2 : MATLAB Function  TreatAsAtomicUnit=on
  Scope : Scope
  Scope1 : Scope
  Scope2 : Scope
  wires:
  Constant2/1 -> MATLAB Function1/2(LoadDemand)
  Constant/1 -> MATLAB Function/4(batteryCapacity)
  Constant3/1 -> MATLAB Function2/2(LoadDemand)
  Constant1/1 -> MATLAB Function/5(timeStep)
  Integrator/1 -> Scope1/1, MATLAB Function1/3(SoC), MATLAB Function2/3(SoC), MATLAB Function/1(currentSoC)
  MATLAB Function2/1(dischargeCurrent) -> MATLAB Function/3(dischargeCurrent)
  MATLAB Function/1(newSoC) -> Integrator/1, Scope/1
  MATLAB Function1/1(chargeCurrent) -> MATLAB Function/2(chargeCurrent)
  PVPower/1 -> MATLAB Function2/1(PVPower), Scope2/1, MATLAB Function1/1(PVPower)

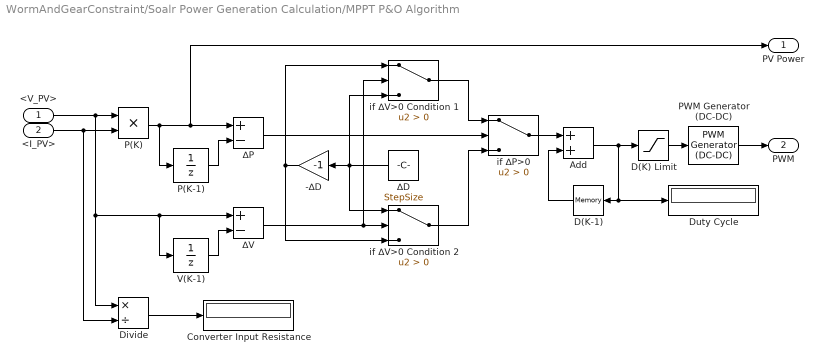
== system WormAndGearConstraint/Soalr Power Generation Calculation/MPPT P&O Algorithm ==
  <V_PV> : Inport
  <I_PV> : Inport  Port=2
  -∆D : Gain  Gain=-1
  Add : Sum
  Converter Input Resistance : Display
  D(K) Limit : Saturate  UpperLimit=1  LowerLimit=0
  D(K-1) : Memory  InitialCondition=0.5  InheritSampleTime=on
  Divide : Product  Inputs=*/
  Duty Cycle : Display
  P(K) : Product
  P(K-1) : UnitDelay  SampleTime=-1  HasFrameUpgradeWarning=on
  PWM Generator (DC-DC) : spsPWMGeneratorDCDCLib/PWM Generator (DC-DC)  Fsw=Fsw  Ts=0
  V(K-1) : UnitDelay  SampleTime=-1  HasFrameUpgradeWarning=on
  if ∆P>0 : Switch  Criteria=u2 > Threshold  SaturateOnIntegerOverflow=off  InputSameDT=off
  if ∆V>0 Condition 1 : Switch  Criteria=u2 > Threshold  SaturateOnIntegerOverflow=off  InputSameDT=off
  if ∆V>0 Condition 2 : Switch  Criteria=u2 > Threshold  SaturateOnIntegerOverflow=off  InputSameDT=off
  ∆D : Constant  Value=StepSize
  ∆P : Sum  Inputs=+-
  ∆V : Sum  Inputs=+-
  PV Power : Outport  VectorParamsAs1DForOutWhenUnconnected=off
  PWM : Outport  Port=2  VectorParamsAs1DForOutWhenUnconnected=off
  wires:
  P(K)/1 -> ∆P/1, PV Power/1, P(K-1)/1
  <I_PV>/1 -> P(K)/2, Divide/2
  if ∆P>0/1 -> Add/1
  if ∆V>0 Condition 1/1 -> if ∆P>0/1
  ∆P/1 -> if ∆P>0/2
  P(K-1)/1 -> ∆P/2
  V(K-1)/1 -> ∆V/2
  ∆V/1 -> if ∆V>0 Condition 2/2, if ∆V>0 Condition 1/2
  <V_PV>/1 -> Divide/1, ∆V/1, V(K-1)/1, P(K)/1
  Add/1 -> D(K) Limit/1, Duty Cycle/1, D(K-1)/1
  if ∆V>0 Condition 2/1 -> if ∆P>0/3
  D(K-1)/1 -> Add/2
  ∆D/1 -> if ∆V>0 Condition 2/1, -∆D/1, if ∆V>0 Condition 1/3
  -∆D/1 -> if ∆V>0 Condition 2/3, if ∆V>0 Condition 1/1
  PWM Generator (DC-DC)/1 -> PWM/1
  Divide/1 -> Converter Input Resistance/1
  D(K) Limit/1 -> PWM Generator (DC-DC)/1

== system WormAndGearConstraint/Soalr Power Generation Calculation/Optical model1 ==
  From2 : From  Commented=on  GotoTag=I2
  From6 : From  Commented=on  GotoTag=V2
  Goto1 : Goto  Commented=on  GotoTag=P2  TagVisibility=global
  MATLAB Function : MATLAB Function  TreatAsAtomicUnit=on
  Product1 : Product  Commented=on
  tag scope: C2=global
  wires:
  MATLAB Function/1(Ir2) -> [C2]
  Product1/1 -> Goto1/1
  From2/1 -> Product1/1
  From6/1 -> Product1/2
  [A2] -> MATLAB Function/2(Incl)
  [S2] -> MATLAB Function/1(S2)

== system WormAndGearConstraint/Soalr Power Generation Calculation/Solar inputs1 ==
  note: Inclination angle zero.
      | As panel follows the SUN
  Inport : Inport
  Inport1 : Inport  Port=2
  1-D Lookup Table1 : Lookup_n-D  NumberOfTableDimensions=1  BreakpointsForDimension1=1:721  Table=zeros(1, 721)  InternalRulePriority=Speed  RndMeth=Simplest
  ANN For Solar Data : Subsystem
      mask help: Function Fitting Neural Network
      mask Display: e = 0.06;c1 = [120 150 230]/255;c2 = ([120 150 230]+0)/383;c3 = ([120 150 230]+128)/383;patch([0 1 1 0],[0 0 1 1],c1);patch([0 1 1 1-e 1-e 0+e],[0 0 1 1-e 0+e 0+e],c2);patch([0 0 1 1-e 0+e 0+e],[0 1 1 1-e 1-e 0+e],c3);plot([0 1 1 0 0],[0 0 1 1 0]);fprintf('NNET');port_label('input',1,' Input');port_label('output',1,'Output ');
  Clock : Clock
  MATLAB Function1 : MATLAB Function  TreatAsAtomicUnit=on
  tag scope: A2=global, S2=global
  wires:
  1-D Lookup Table1/1 -> [A2]
  Clock/1 -> 1-D Lookup Table1/1
  MATLAB Function1/1(output) -> ANN For Solar Data/1(Input)
  ANN For Solar Data/1(Output) -> [S2]
  Inport/1 -> MATLAB Function1/1(lat)
  Inport1/1 -> MATLAB Function1/2(lon)

== system WormAndGearConstraint/Solar Array/ANN For Solar Data ==
  Input : Inport  PortDimensions=5
      mask Display: e = 0.06;c1 = [120 230 180]/255;c2 = ([120 230 180]+0)/(256+128);c3 = ([120 230 180]+128)/(256+128);patch([0 1 1 0],[0 0 1 1],c1);patch([0 1 1 1-e 1-e 0+e],[0 0 1 1-e 0+e 0+e],c2);patch([0 0 1 1-e 0+e 0+e],[0 1 1 1-e 1-e 0+e],c3);plot([0 1 1 0 0],[0 0 1 1 0]);
  Layer 1 : Subsystem
      mask Display: e = 0.06;c1 = [120 150 230]/255;c2 = ([120 150 230]+0)/383;c3 = ([120 150 230]+128)/383;patch([0 1 1 0],[0 0 1 1],c1);patch([0 1 1 1-e 1-e 0+e],[0 0 1 1-e 0+e 0+e],c2);patch([0 0 1 1-e 0+e 0+e],[0 1 1 1-e 1-e 0+e],c3);plot([0 1 1 0 0],[0 0 1 1 0]);
  Layer 2 : Subsystem
      mask Display: e = 0.06;c1 = [120 150 230]/255;c2 = ([120 150 230]+0)/383;c3 = ([120 150 230]+128)/383;patch([0 1 1 0],[0 0 1 1],c1);patch([0 1 1 1-e 1-e 0+e],[0 0 1 1-e 0+e 0+e],c2);patch([0 0 1 1-e 0+e 0+e],[0 1 1 1-e 1-e 0+e],c3);plot([0 1 1 0 0],[0 0 1 1 0]);
  Process Input 1 : Subsystem
      mask Display: e = 0.06;c1 = [120 150 230]/255;c2 = ([120 150 230]+0)/383;c3 = ([120 150 230]+128)/383;patch([0 1 1 0],[0 0 1 1],c1);patch([0 1 1 1-e 1-e 0+e],[0 0 1 1-e 0+e 0+e],c2);patch([0 0 1 1-e 0+e 0+e],[0 1 1 1-e 1-e 0+e],c3);plot([0 1 1 0 0],[0 0 1 1 0]);
  Process Output 1 : Subsystem
      mask Display: e = 0.06;c1 = [120 150 230]/255;c2 = ([120 150 230]+0)/383;c3 = ([120 150 230]+128)/383;patch([0 1 1 0],[0 0 1 1],c1);patch([0 1 1 1-e 1-e 0+e],[0 0 1 1-e 0+e 0+e],c2);patch([0 0 1 1-e 0+e 0+e],[0 1 1 1-e 1-e 0+e],c3);plot([0 1 1 0 0],[0 0 1 1 0]);
  Output : Outport  InitialOutput=0
      mask Display: e = 0.06;c1 = [120 230 180]/255;c2 = ([120 230 180]+0)/(256+128);c3 = ([120 230 180]+128)/(256+128);patch([0 1 1 0],[0 0 1 1],c1);patch([0 1 1 1-e 1-e 0+e],[0 0 1 1-e 0+e 0+e],c2);patch([0 0 1 1-e 0+e 0+e],[0 1 1 1-e 1-e 0+e],c3);plot([0 1 1 0 0],[0 0 1 1 0]);
  wires:
  Input/1 -> Process Input 1/1(x)
  Process Output 1/1(y) -> Output/1
  Process Input 1/1(p) -> Layer 1/1("p{1}")
  Layer 1/1("a{1}") -> [feedback1]
  [feedback1] -> Layer 2/1("a{1} ")
  Layer 2/1("a{2}") -> Process Output 1/1(a)

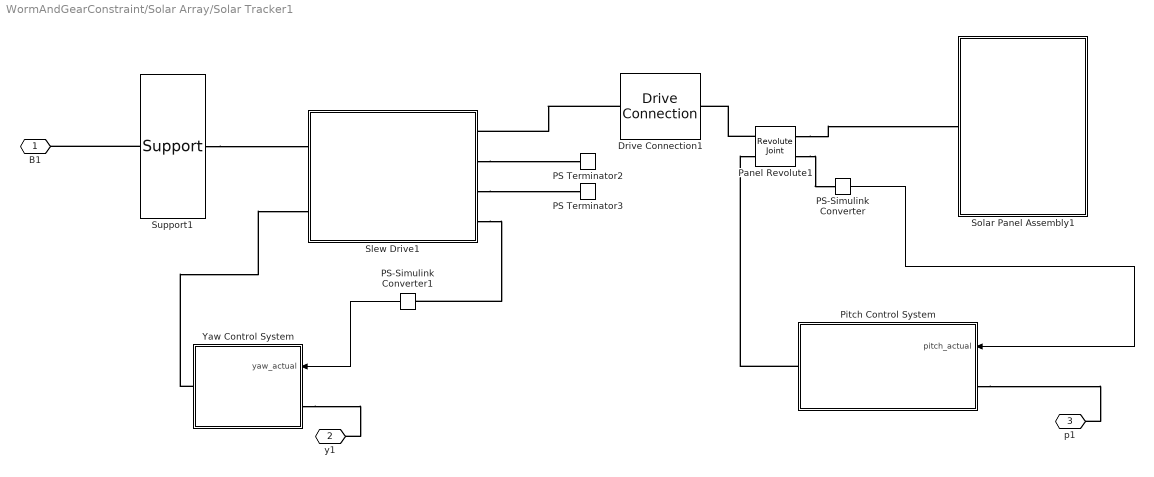
== system WormAndGearConstraint/Solar Array/Solar Tracker1 ==
  Drive Connection1 : WormAndGearConstraintLibrary/Drive Connection  connRadius=driveconn.connectionRadius  connThickness=driveconn.connectionThickness  connLength=driveconn.connectionLength  bracketWidth=driveconn.bracketWidthHeight  bracketThickness=driveconn.bracketThickness  holeRadius=driveconn.holeRadius  holeOffset=driveconn.holeOffset  baseThickness=driveconn.baseThickness  rho=driveconn.density  color=driveconn.color
      settings: LibrarySourceBlock=sm_solar_tracker_lib/Drive Connection
  PS Terminator2 : fl_lib/Physical Signals/Sinks/PS Terminator
  PS Terminator3 : fl_lib/Physical Signals/Sinks/PS Terminator
  PS-Simulink Converter : nesl_utility/PS-Simulink Converter  PhysicalDomain=network_engine_domain  SubClassName=ps_output  LeftPortType=input  RightPortType=output  PseudoPeriodic=off  Frequencies=[]  VectorFormat=inherit  Unit=inherit  AffineConversion=off
  PS-Simulink Converter1 : nesl_utility/PS-Simulink Converter  PhysicalDomain=network_engine_domain  SubClassName=ps_output  LeftPortType=input  RightPortType=output  PseudoPeriodic=off  Frequencies=[]  VectorFormat=inherit  Unit=inherit  AffineConversion=off
  Panel Revolute1 : sm_lib/Joints/Revolute Joint  JointMode=Normal  CompositeWrenchDir=FollowerOnBase  CompositeWrenchFrame=BaseFrame  SenseConstraintForce=off  SenseConstraintTorque=off  SenseTotalForce=off  SenseTotalTorque=off  PositionTargetSpecify=on  PositionTargetPriority=High  PositionTargetValue=panelrevolute.q0  PositionTargetValueUnits=deg  VelocityTargetSpecify=off  VelocityTargetPriority=High  VelocityTargetValue=0  VelocityTargetValueUnits=deg/s  EquilibriumPosition=0  EquilibriumPositionUnits=deg  SpringStiffness=0  SpringStiffnessUnits=N*m/deg  DampingCoefficient=0  DampingCoefficientUnits=N*m/(deg/s)  LowerLimitSpecify=off  LowerLimitBound=-90  LowerLimitBoundUnits=deg  LowerLimitStiffness=1e4  LowerLimitStiffnessUnits=N*m/deg  LowerLimitDamping=10  LowerLimitDampingUnits=N*m/(deg/s)  LowerLimitTransitionRegionWidth=0.1  LowerLimitTransitionRegionWidthUnits=deg  UpperLimitSpecify=off  UpperLimitBound=90  UpperLimitBoundUnits=deg  UpperLimitStiffness=1e4  UpperLimitStiffnessUnits=N*m/deg  UpperLimitDamping=10  UpperLimitDampingUnits=N*m/(deg/s)  UpperLimitTransitionRegionWidth=0.1  UpperLimitTransitionRegionWidthUnits=deg  TorqueActuationMode=ComputedTorque  MotionActuationMode=InputMotion  SensePosition=on  SenseVelocity=off  SenseAcceleration=off  SenseTorqueForce=off  SenseLowerLimitTorqueForce=off  SenseUpperLimitTorqueForce=off
  Pitch Control System : Subsystem
  Slew Drive1 : Subsystem  AncestorBlock=WormAndGearConstraintLibrary/Slew Drive  mask(Slew Drive){wormLeadAngle=slewdrive.wormLeadAngle, wormLength=slewdrive.wormLength, gearOuterRadius=slewdrive.gearOuterRadius, gearInnerRadius=slewdrive.gearInnerRadius, gearExposedRadius=slewdrive.gearExposedRadius, ratio=slewdrive.ratio, housingThickness=slewdrive.housingThickness, bWormRevolute=slewdrive.wormRevoluteDamping, wormRho=slewdrive.wormDensity, gearRho=slewdrive.gearDensity, housingRho=slewdrive.housingDensity, wormColor=slewdrive.wormColor, gearColor=slewdrive.gearColor, housingColor=slewdrive.housingColor, housingOpacity=slewdrive.housingOpacity}
      mask prompts: wormLeadAngle "Worm Lead Angle (deg)"; wormLength "Worm Length (m)"; gearOuterRadius "Gear Outer Radius (m)"; gearInnerRadius "Gear Inner Radius (m)"; gearExposedRadius "Gear Exposed Radius (m)"; ratio "Ratio (Ng / Nw)"; housingThickness "Housing Thickness (m)"; bWormRevolute "Worm Revolute Damping (Nm/(deg/s))"; wormRho "Worm Density (kg/m^3)"; gearRho "Gear Density (kg/m^3)"; housingRho "Housing Density (kg/m3)"; wormColor "Worm Color [r g b]"; gearColor "Gear Color [r g b]"; housingColor "Housing Color [r g b]"; housingOpacity "Housing Opacity"
      mask help:
      | This block models the slew drive of the solar tracker.
      |
      | Port B corresponds to the base face of the housing aligned with the gear axis. Port T corresponds to the center of the top face of the gear.
      |
      | Input port q specifies the motion actuation signal of the gear revolute. Output port w corresponds to the angular velocity of the worm revolute. Output port t corresponds to the automatically computed actuation torque at the worm revolute necessary to achieve the desired motion signal of the gear revolute.
      mask init:
      | % Worm Properties
      | wormRadius            = gearOuterRadius / (ratio * tand(wormLeadAngle));
      | wormNonThreadedRadius = 0.4*wormRadius;
      | 
      | wormThreadedLength    = 0.4*wormLength;
      | wormNonThreadedLength = 0.5*(wormLength - wormThreadedLength);
      | 
      | wormHoleRadius = 0.5*wormNonThreadedRadius;
      | 
      | wormThreadedThickness    = wormRadius - wormHoleRadius;
      | wormNonThreadedThickness = wormNonThreadedRadius - wormHoleRadius;
      | 
      | wormSliceColor      = 0.75*wormColor;
      | wormSliceProportion = 0.25;
      | 
      | % Worm Offsets
      | wormLeftOffset  = [-0.5*wormLength gearOuterRadius+wormRadius 0];
      | wormRightOffset = [ 0.5*wormLength gearOuterRadius+wormRadius 0];
      | 
      | % Gear Properties
      | gearLength         = wormRadius;
      | gearThickness      = gearOuterRadius - gearInnerRadius;
      | gearSliceThickness = 0.1*gearOuterRadius;
      | gearSliceColor     = 0.75*gearColor;
      | 
      | % Housing Dimensions
      | housingRadTol = 0.05*gearOuterRadius;
      | sideDepth     = 2*wormRadius + 2*housingRadTol;
      | 
      | % Housing Base Vertices
      | baseVertex1_x = 0;
      | baseVertex2_x = housingThickness + housingRadTol + 2*wormRadius;
      | baseVertex3_x = baseVertex2_x + gearOuterRadius;
      | baseVertex4_x = baseVertex3_x + gearOuterRadius + housingRadTol + housingThickness;
      | 
      | baseVertex1_y = -0.5*wormLength - housingThickness;
      | baseVertex2_y = baseVertex1_y;
      | baseVertex3_y = -gearOuterRadius - housingRadTol - housingThickness;
      | baseVertex4_y = baseVertex3_y;
      | 
      | baseVertices = [...
      |   baseVertex1_x  baseVertex1_y;...
      |   baseVertex2_x  baseVertex2_y;...
      |   baseVertex3_x  baseVertex3_y;...
      |   baseVertex4_x  baseVertex4_y;...
      |   baseVertex4_x -baseVertex4_y;...
      |   baseVertex3_x -baseVertex3_y;...
      |   baseVertex2_x -baseVertex2_y;...
      |   baseVertex1_x -baseVertex1_y];
      | 
      | baseVertex1_R = 0.5*wormRadius + housingRadTol + housingThickness;
      | baseVertex4_R = gearOuterRadius + housingRadTol + housingThickness;
      | baseVertex5_R = baseVertex4_R;
      | baseVertex8_R = baseVertex1_R;
      | 
      | baseVerticesR = [baseVertex1_R baseVertex4_R baseVertex5_R baseVertex8_R];
      |   
      | baseVertices = simmechanics.demohelpers.round_corners(...
      |   baseVertices, [1 4 5 8], baseVerticesR, 20);
      | 
      | % Housing Side Vertices
      | sideVertices = [...
      |   baseVertex1_x+housingThickness  baseVertex1_y+housingThickness;...
      |   baseVertex2_x                   baseVertex2_y+housingThickness;...
      |   baseVertex3_x                   baseVertex3_y+housingThickness;...
      |   baseVertex4_x-housingThickness  baseVertex4_y+housingThickness;...
      |   baseVertex4_x-housingThickness -baseVertex4_y-housingThickness;...
      |   baseVertex3_x                  -baseVertex3_y-housingThickness;...
      |   baseVertex2_x                  -baseVertex2_y-housingThickness;...
      |   baseVertex1_x+housingThickness -baseVertex1_y-housingThickness];
      | 
      | sideVertex1_R = 0.5*wormRadius + housingRadTol;
      | sideVertex4_R = gearOuterRadius + housingRadTol;
      | sideVertex5_R = sideVertex4_R;
      | sideVertex8_R = sideVertex1_R;
      | 
      | sideVerticesR = [sideVertex1_R sideVertex4_R sideVertex5_R sideVertex8_R];
      | 
      | sideVertices = simmechanics.demohelpers.round_corners(...
      |   sideVertices, [1 4 5 8], sideVerticesR, 20);
      | 
      | sideVertices = flipud(sideVertices);
      | sideVertices(end+1,:) = sideVertices(1,:);
      | 
      | sideVertices = [sideVertices; baseVertices(end,:); baseVertices];
      | 
      | % Housing Top Vertices
      | topHoleOffset = housingThickness + housingRadTol + 2*wormRadius + gearOuterRadius;
      | 
      | topHoleTheta = linspace(pi, -pi, 40);
      | topVertices = [gearExposedRadius*cos(topHoleTheta)+topHoleOffset;...
      |                gearExposedRadius*sin(topHoleTheta)]';
      | 
      | topVertices = [topVertices; 0 0; baseVertices; 0 0];
      | 
      | % Housing Offsets
      | housingOffset        = topHoleOffset;
      | housingTopBaseOffset = 0.5*sideDepth + 0.5*housingThickness;
      | baseOffset           = [topHoleOffset 0 -0.5*housingThickness];
      settings: LibrarySourceBlock=sm_solar_tracker_lib/Slew Drive
      mask DialogControl Tab1 Prompt: Dimensions
      mask DialogControl Tab2 Prompt: Internal Mechanics
      mask DialogControl Tab3 Prompt: Material Properties
      mask Display:
      | image(fullfile('WormAndGearConstraintSupport','Images','SlewDrive.png'));
      | port_label('lconn',1,'B');
      | port_label('lconn',2,'q');
      | port_label('rconn',1,'T');
      | port_label('rconn',2,'w');
      | port_label('rconn',3,'t');
  Solar Panel Assembly1 : Subsystem
      mask Display:
      | image(fullfile('WormAndGearConstraintSupport','Images','SolarPanel.png'));
      | port_label('lconn',1,'H');
  Support1 : WormAndGearConstraintLibrary/Support  columnRadius=support.columnRadius  columnThickness=support.columnThickness  columnHeight=support.columnHeight  baseWidth=support.baseWidth  baseThickness=support.baseThickness  rho=support.density  color=support.color
      settings: LibrarySourceBlock=sm_solar_tracker_lib/Support
  Yaw Control System : Subsystem
  B1 : PMIOPort  Side=Left
  y1 : PMIOPort  Port=2  Side=Left
  p1 : PMIOPort  Port=3  Side=Left
  wires:
  PS-Simulink Converter1/1 -> Yaw Control System/1(yaw_actual)
  PS-Simulink Converter/1 -> Pitch Control System/1(pitch_actual)
  connections:
  Yaw Control System/LConn1 -- y1/RConn1
  Yaw Control System/RConn1 -- Slew Drive1/LConn2
  Drive Connection1/LConn1 -- Slew Drive1/RConn1
  Panel Revolute1/LConn1 -- Drive Connection1/RConn1
  Slew Drive1/RConn4 -- PS-Simulink Converter1/LConn1
  Support1/RConn1 -- Slew Drive1/LConn1
  Panel Revolute1/RConn2 -- PS-Simulink Converter/LConn1
  Support1/LConn1 -- B1/RConn1
  Slew Drive1/RConn3 -- PS Terminator3/LConn1
  Slew Drive1/RConn2 -- PS Terminator2/LConn1
  Panel Revolute1/RConn1 -- Solar Panel Assembly1/LConn1
  Pitch Control System/RConn1 -- Panel Revolute1/LConn2
  Pitch Control System/LConn1 -- p1/RConn1
